simulink library "Gravity_ul"  (R2020a)
settings: Solver=VariableStepAuto  StartTime=0.0  StopTime=10.0  RelTol=1e-3
undefined symbols (not defined in the file): Env
settings Model: Creator=bunce  LastModifiedBy=bunce

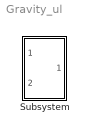
== system Gravity_ul ==
  Subsystem : Subsystem

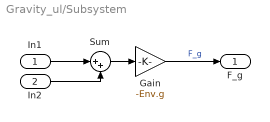
== system Gravity_ul/Subsystem ==
  In1 : Inport
  In2 : Inport  Port=2
  Gain : Gain  Gain=-Env.g
  Sum : Sum  Inputs=|++
  F_g : Outport
  wires:
  In2/1 -> Sum/2
  Sum/1 -> Gain/1
  Gain/1 -> F_g/1  "F_g"
  In1/1 -> Sum/1
